simulink model "scattering_force_pos"  (R2022b)
settings: Solver=VariableStepAuto  StartTime=0.0  StopTime=20  RelTol=1e-3
values from neighbouring files (symbols this model uses):
  A = 2    [scattering_params.m]    (also in scattering_params_force_pos.m = 3; scattering_params_pos_pos.m = 1)
  b = 1    [scattering_params.m]    (also in scattering_params_force_pos.m = 40; scattering_params_pos_pos.m = 100)
  Be = 100    [scattering_params.m]    (also in scattering_params_force_pos.m; scattering_params_pos_pos.m)
  Bh = 1.5    [scattering_params.m]    (also in scattering_params_force_pos.m = 1; scattering_params_pos_pos.m = 1)
  Bm = 20*0.8    (= 16)    [scattering_params.m]
  Bs = 80    [scattering_params.m]    (also in scattering_params_force_pos.m = 10)
  Fc = 1    [scattering_params.m]    (also in scattering_params_force_pos.m = 0.25; scattering_params_pos_pos.m = 0.25)
  Flp = 5    [scattering_params.m]    (also in scattering_params_force_pos.m = 0.5; scattering_params_pos_pos.m = 0.5)
  Jh = 1    [scattering_params.m]    (also in scattering_params_force_pos.m; scattering_params_pos_pos.m)
  Ke = 200    [scattering_params.m]    (also in scattering_params_force_pos.m; scattering_params_pos_pos.m)
  Km = 10*1    (= 10)    [scattering_params.m]
  Ks = 100    [scattering_params.m]    (also in scattering_params_force_pos.m)
  Mm = 0.5    [scattering_params.m]    (also in scattering_params_force_pos.m; scattering_params_pos_pos.m)
  Ms = 2    [scattering_params.m]    (also in scattering_params_force_pos.m; scattering_params_pos_pos.m)
  Ph = 10    [scattering_params.m]    (also in scattering_params_force_pos.m; scattering_params_pos_pos.m)
  scattering_filter_freq = 10    [scattering_params.m]    (also in scattering_params_force_pos.m; scattering_params_pos_pos.m = 100)
  time_delay = 0    [scattering_params.m]
  xe = 5    [scattering_params.m]    (also in scattering_params_force_pos.m = 2; scattering_params_pos_pos.m = 2)
settings Model: Creator=Manu  LastModifiedBy=Manu

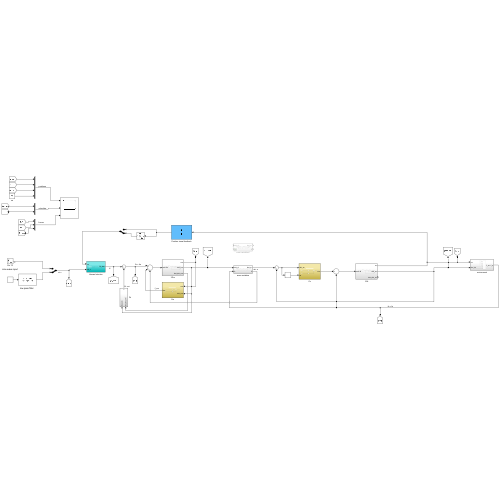
[thumbnail: Simulink's stored preview of the top-level diagram]
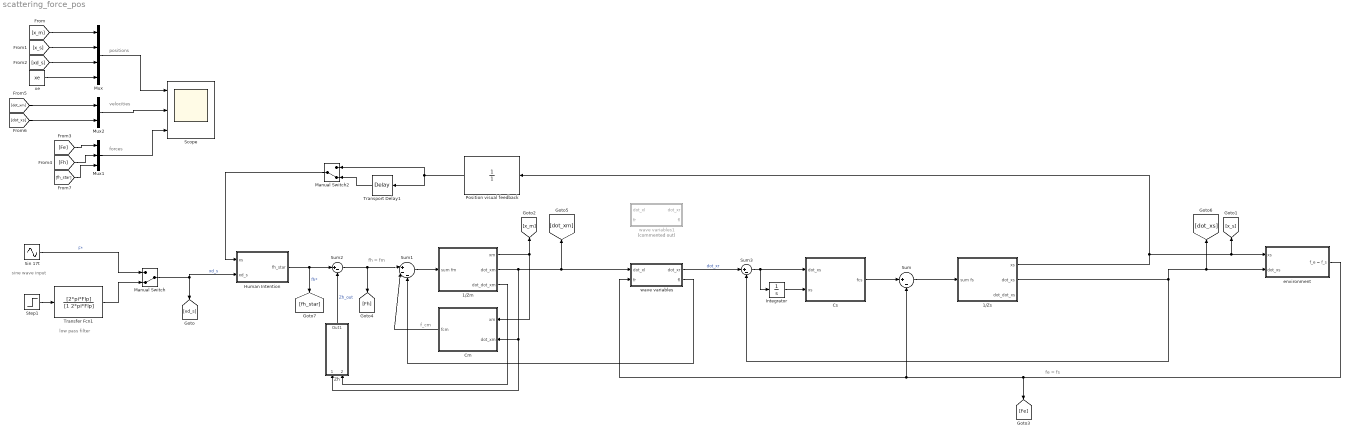
== system scattering_force_pos ==
  note: positions
  note: fe = fs
  note: f_cm
  note: fh = fm
  note: sine wave input
  note: low pass filter
  note: forces
  note: velocities
  1/Zm : Subsystem
  1/Zs : Subsystem
  Cm : Subsystem
  Cs : Subsystem
  Human Intention : Subsystem
  Integrator : Integrator
  Manual Switch : ManualSwitch  CurrentSetting=0
  Manual Switch2 : ManualSwitch  CurrentSetting=0
  Mux : Mux
  Mux1 : Mux  Inputs=3
  Mux2 : Mux  Inputs=2
  Position visual feedback : TransferFcn  Denominator=[1]
  Scope : Scope  NumInputPorts=3
  Sin 17t : Sin  Amplitude=A  Frequency=2*pi*Fc  SampleTime=0
  Step1 : Step  Time=0.5  After=A  SampleTime=0
  Sum : Sum  Inputs=|+-
  Sum1 : Sum  Inputs=|+--
  Sum2 : Sum  Inputs=|+-
  Sum3 : Sum  Inputs=|+-
  Transfer Fcn1 : TransferFcn  Numerator=[2*pi*Flp]  Denominator=[1 2*pi*Flp]
  Transport Delay1 : TransportDelay  DelayTime=time_delay
  Zh : Subsystem
  environment : Subsystem
  wave variables : Subsystem
  wave variables1 : Subsystem  Commented=on
  xe : Constant  Value=xe
  wires:
  1/Zm/2(dot_xm) -> wave variables/1(dot_xl), [dot_xm], Cm/2(dot_xm), Zh/1(dot_xm)
  1/Zm/1(xm) -> Cm/1(xm), [x_m]
  Manual Switch/1 -> [xd_s], Human Intention/2(xd_s)  "xd_s"
  Zh/1(Out1) -> Sum2/2  "Zh_out"
  Sin 17t/1 -> Manual Switch/1  "F*"
  1/Zm/3(dot_dot_xm) -> Zh/2(dot_dot_xm)
  Human Intention/1(fh_star) -> Sum2/1, [fh_star]  "fh*"
  Transfer Fcn1/1 -> Manual Switch/2
  Step1/1 -> Transfer Fcn1/1
  Sum2/1 -> Sum1/1, [Fh]
  Sum1/1 -> 1/Zm/1(sum fm)
  Sum/1 -> 1/Zs/1(sum fs)
  1/Zs/2(dot_xs) -> [dot_xs], environment/2(dot_xs), Sum3/2
  1/Zs/1(xs) -> [x_s], environment/1(xs), Position visual feedback/1
  environment/1(f_e = f_s) -> wave variables/2(fr), Sum/2, [Fe]
  Mux/1 -> Scope/1
  [x_s] -> Mux/2
  [xd_s] -> Mux/3
  xe/1 -> Mux/4
  [x_m] -> Mux/1
  Mux1/1 -> Scope/3
  [Fe] -> Mux1/1
  [Fh] -> Mux1/2
  [dot_xs] -> Mux2/2
  [dot_xm] -> Mux2/1
  Mux2/1 -> Scope/2
  [fh_star] -> Mux1/3
  Transport Delay1/1 -> Manual Switch2/2
  Position visual feedback/1 -> Transport Delay1/1, Manual Switch2/1
  Manual Switch2/1 -> Human Intention/1(xs)
  Sum3/1 -> Cs/1(dot_xs), Integrator/1
  Integrator/1 -> Cs/2(xs)
  Cs/1(fcs) -> Sum/1
  Cm/1(fcm) -> Sum1/2
  wave variables/1(dot_xr) -> Sum3/1  "dot_xr"
  wave variables/2(fl) -> Sum1/3

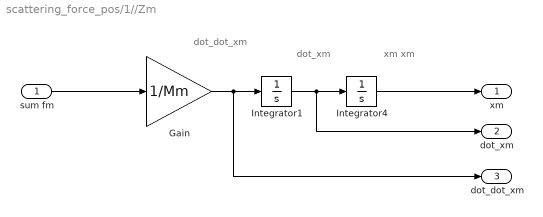
== system scattering_force_pos/1//Zm ==
  note: dot_dot_xm
  note: dot_xm
  note: xm
      | xm
  sum fm : Inport
  Gain : Gain  Gain=1/Mm
  Integrator1 : Integrator
  Integrator4 : Integrator
  xm : Outport
  dot_xm : Outport  Port=2
  dot_dot_xm : Outport  Port=3
  wires:
  sum fm/1 -> Gain/1
  Gain/1 -> dot_dot_xm/1, Integrator1/1
  Integrator4/1 -> xm/1
  Integrator1/1 -> dot_xm/1, Integrator4/1

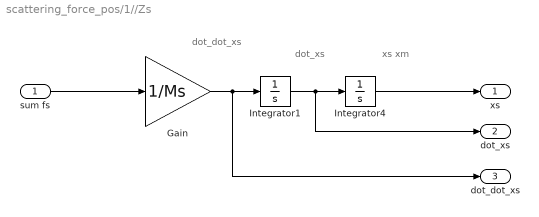
== system scattering_force_pos/1//Zs ==
  note: dot_dot_xs
  note: dot_xs
  note: xs
      | xm
  sum fs : Inport
  Gain : Gain  Gain=1/Ms
  Integrator1 : Integrator
  Integrator4 : Integrator
  xs : Outport
  dot_xs : Outport  Port=2
  dot_dot_xs : Outport  Port=3
  wires:
  sum fs/1 -> Gain/1
  Gain/1 -> dot_dot_xs/1, Integrator1/1
  Integrator4/1 -> xs/1
  Integrator1/1 -> dot_xs/1, Integrator4/1

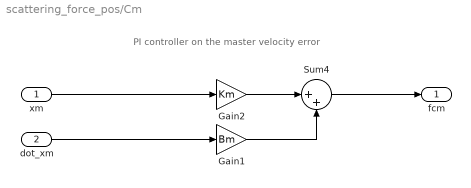
== system scattering_force_pos/Cm ==
  note: PI controller on the master velocity error
  xm : Inport
  dot_xm : Inport  Port=2
  Gain1 : Gain  Gain=Bm
  Gain2 : Gain  Gain=Km
  Sum4 : Sum  Inputs=|++
  fcm : Outport
  wires:
  Sum4/1 -> fcm/1
  xm/1 -> Gain2/1
  Gain2/1 -> Sum4/1
  dot_xm/1 -> Gain1/1
  Gain1/1 -> Sum4/2

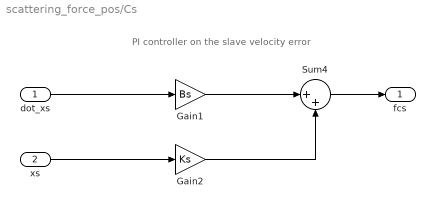
== system scattering_force_pos/Cs ==
  note: PI controller on the slave velocity error
  dot_xs : Inport
  xs : Inport  Port=2
  Gain1 : Gain  Gain=Bs
  Gain2 : Gain  Gain=Ks
  Sum4 : Sum  Inputs=|++
  fcs : Outport
  wires:
  Sum4/1 -> fcs/1
  xs/1 -> Gain2/1
  Gain2/1 -> Sum4/2
  dot_xs/1 -> Gain1/1
  Gain1/1 -> Sum4/1

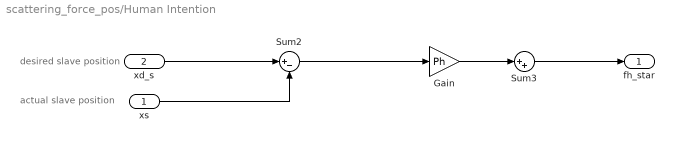
== system scattering_force_pos/Human Intention ==
  note: actual slave position
  note: desired slave position
  xs : Inport
  xd_s : Inport  Port=2
  Gain : Gain  Gain=Ph
  Sum2 : Sum  Inputs=|+-
  Sum3 : Sum  Inputs=|++
  fh_star : Outport
  wires:
  xs/1 -> Sum2/2
  Sum2/1 -> Gain/1
  Gain/1 -> Sum3/1
  Sum3/1 -> fh_star/1
  xd_s/1 -> Sum2/1

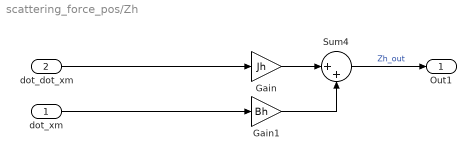
== system scattering_force_pos/Zh ==
  dot_xm : Inport
  dot_dot_xm : Inport  Port=2
  Gain : Gain  Gain=Jh
  Gain1 : Gain  Gain=Bh
  Sum4 : Sum  Inputs=|++
  Out1 : Outport
  wires:
  dot_dot_xm/1 -> Gain/1
  Gain1/1 -> Sum4/2
  Gain/1 -> Sum4/1
  Sum4/1 -> Out1/1  "Zh_out"
  dot_xm/1 -> Gain1/1

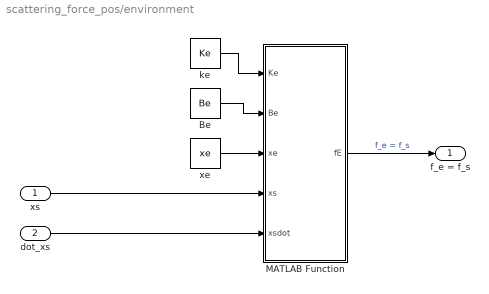
== system scattering_force_pos/environment ==
  xs : Inport
  dot_xs : Inport  Port=2
  Be : Constant  Value=Be
  MATLAB Function : MATLAB Function  TreatAsAtomicUnit=on
  ke : Constant  Value=Ke
  xe : Constant  Value=xe
  f_e = f_s : Outport
  wires:
  MATLAB Function/1(fE) -> f_e = f_s/1  "f_e = f_s"
  xs/1 -> MATLAB Function/4(xs)
  xe/1 -> MATLAB Function/3(xe)
  dot_xs/1 -> MATLAB Function/5(xsdot)
  ke/1 -> MATLAB Function/1(Ke)
  Be/1 -> MATLAB Function/2(Be)

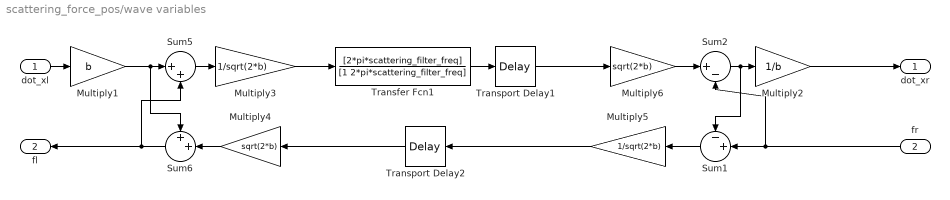
== system scattering_force_pos/wave variables ==
  dot_xl : Inport
  fr : Inport  Port=2
  Multiply1 : Gain  Gain=b
  Multiply2 : Gain  Gain=1/b
  Multiply3 : Gain  Gain=1/sqrt(2*b)
  Multiply4 : Gain  Gain=sqrt(2*b)
  Multiply5 : Gain  Gain=1/sqrt(2*b)
  Multiply6 : Gain  Gain=sqrt(2*b)
  Sum1 : Sum  Inputs=-+|
  Sum2 : Sum  Inputs=|+-
  Sum5 : Sum  Inputs=|++
  Sum6 : Sum  Inputs=++|
  Transfer Fcn1 : TransferFcn  Numerator=[2*pi*scattering_filter_freq]  Denominator=[1 2*pi*scattering_filter_freq]
  Transport Delay1 : TransportDelay  DelayTime=time_delay
  Transport Delay2 : TransportDelay  DelayTime=time_delay
  dot_xr : Outport
  fl : Outport  Port=2
  wires:
  Multiply3/1 -> Transfer Fcn1/1
  Transfer Fcn1/1 -> Transport Delay1/1
  Sum6/1 -> fl/1, Sum5/2
  Multiply4/1 -> Sum6/2
  Multiply1/1 -> Sum6/1, Sum5/1
  Transport Delay2/1 -> Multiply4/1
  Sum5/1 -> Multiply3/1
  dot_xl/1 -> Multiply1/1
  Sum2/1 -> Sum1/1, Multiply2/1
  Multiply6/1 -> Sum2/1
  Multiply5/1 -> Transport Delay2/1
  Transport Delay1/1 -> Multiply6/1
  Sum1/1 -> Multiply5/1
  fr/1 -> Sum2/2, Sum1/2
  Multiply2/1 -> dot_xr/1

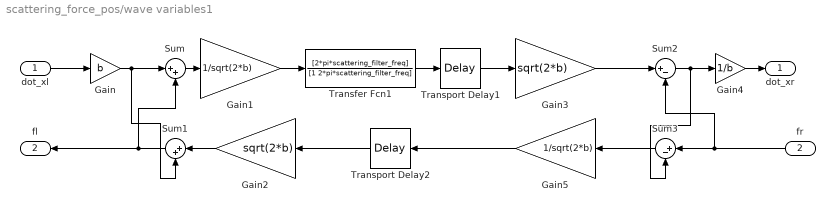
== system scattering_force_pos/wave variables1 ==
  dot_xl : Inport
  fr : Inport  Port=2
  Gain : Gain  Gain=b
  Gain1 : Gain  Gain=1/sqrt(2*b)
  Gain2 : Gain  Gain=sqrt(2*b)
  Gain3 : Gain  Gain=sqrt(2*b)
  Gain4 : Gain  Gain=1/b
  Gain5 : Gain  Gain=1/sqrt(2*b)
  Sum : Sum  Inputs=|++
  Sum1 : Sum  Inputs=|++
  Sum2 : Sum  Inputs=|+-
  Sum3 : Sum  Inputs=|+-
  Transfer Fcn1 : TransferFcn  Numerator=[2*pi*scattering_filter_freq]  Denominator=[1 2*pi*scattering_filter_freq]
  Transport Delay1 : TransportDelay  DelayTime=time_delay
  Transport Delay2 : TransportDelay  DelayTime=time_delay
  dot_xr : Outport
  fl : Outport  Port=2
  wires:
  Sum2/1 -> Sum3/2, Gain4/1
  Gain/1 -> Sum1/2, Sum/1
  Sum/1 -> Gain1/1
  Gain2/1 -> Sum1/1
  fr/1 -> Sum2/2, Sum3/1
  Sum3/1 -> Gain5/1
  Gain3/1 -> Sum2/1
  dot_xl/1 -> Gain/1
  Gain4/1 -> dot_xr/1
  Sum1/1 -> fl/1, Sum/2
  Gain5/1 -> Transport Delay2/1
  Gain1/1 -> Transfer Fcn1/1
  Transport Delay1/1 -> Gain3/1
  Transport Delay2/1 -> Gain2/1
  Transfer Fcn1/1 -> Transport Delay1/1

== matlab function scattering_force_pos/environment/MATLAB Function ==
  data: Ke input; fE output; Be input; xe input; xs input; xsdot input
function fE = environment(Ke, Be, xe, xs, xsdot)
    if xs > xe
        fE = Ke * (xs - xe) + Be * xsdot; % Plot both contributions Ke and Be
    else
        fE = 0;
    end
end
